simulink model "spwm_single_phase"  (R2020a)
settings: Solver=VariableStepAuto  StartTime=0.0  StopTime=1  RelTol=1e-3
libraries: simulink x16, powerlib_meascontrol x1, powerlib x1
settings Model: Creator=Junaed  LastModifiedBy=Junaed

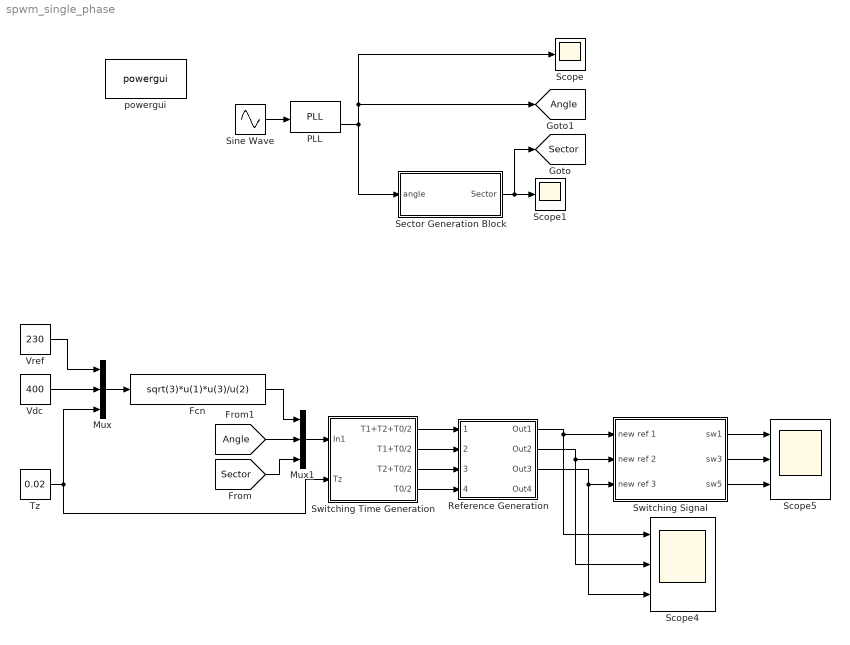
== system spwm_single_phase ==
  Fcn : Fcn  Expr=sqrt(3)*u(1)*u(3)/u(2)
  Mux : Mux  Inputs=3
  Mux1 : Mux  Inputs=3
  PLL : powerlib_meascontrol/PLL/PLL  Fmin=45  Par_Init=[0, 60]  ParK=[180, 3200, 1]  TcD=1e-4  MaxRateChangeFreq=12  FilterCutOffFreq=25  Ts=0  AGC=on
      settings: SourceProductBaseCode=PS
  Reference Generation : Subsystem
  Scope : Scope
  Scope1 : Scope
  Scope4 : Scope  NumInputPorts=3
  Scope5 : Scope  NumInputPorts=3
  Sector Generation Block : Subsystem
  Sine Wave : Sin  Frequency=2*pi*50  SampleTime=0
  "Switching Signal " : Subsystem
  Switching Time Generation : Subsystem
  Tz : Constant  Value=0.02
  Vdc : Constant  Value=400
  Vref : Constant  Value=230
  powergui : powerlib/powergui  Priority=1  SimulationMode=Continuous  SampleTime=50e-6  frequency=60  Iterations=50  frequencyindice=60  Pbase=100e6  ErrMax=1e-4  UnitsV=kV  UnitsW=MW  buscounter=0  FunctionMessages=off  echomessages=off  EnableUseOfTLC=off  CurrentSourceSwitches=off  DisableSnubberDevices=off  DisableRonSwitches=off  DisableVfSwitches=off  DisplayEquations=off  AutomaticDiscreteSolvers=off  SolverType=Tustin/Backward Euler (TBE)  Interpol=off  ExternalGateDelay=off  methode=off  Ts=100  x0status=blocks  SPID=on  SwTol=0  HookPort=off  NonlinearTolerance=1e-4  nMaxIteration=100  ContinueOnMaxIteration=off  RestoreLinks=warning  ResistiveCurrentMeasurement=off  Frange=[0:2:500]  Ylog=off  Xlog=on  ShowGrid=off  save=off  variable=ZData  structure=0  ZoomFFT=off  StartTime=0.0  cycles=1  DisplayStyle=1  fundamental=60  FreqAxis=off  MaxFrequency=1000  frequencyindicesteady=1  RmsSteady=1  display=off
  tag scope: Angle=global, Sector=global
  wires:
  Vref/1 -> Mux/1
  Vdc/1 -> Mux/2
  Tz/1 -> Switching Time Generation/2(Tz), Mux/3
  Mux/1 -> Fcn/1
  Fcn/1 -> Mux1/1
  [Angle] -> Mux1/2
  [Sector] -> Mux1/3
  "Switching Signal "/1(sw1) -> Scope5/1
  "Switching Signal "/2(sw3) -> Scope5/2
  "Switching Signal "/3(sw5) -> Scope5/3
  Mux1/1 -> Switching Time Generation/1(In1)
  Reference Generation/2(Out2) -> "Switching Signal "/2(new ref 2), Scope4/2
  Reference Generation/1(Out1) -> "Switching Signal "/1(new ref 1), Scope4/1
  Switching Time Generation/1(T1+T2+T0/2) -> Reference Generation/1(1)
  Switching Time Generation/2(T1+T0/2) -> Reference Generation/2(2)
  Switching Time Generation/3(T2+T0/2) -> Reference Generation/3(3)
  Switching Time Generation/4(T0/2) -> Reference Generation/4(4)
  PLL/2 -> Sector Generation Block/1(angle), Scope/1, [Angle]
  Sine Wave/1 -> PLL/1
  Sector Generation Block/1(Sector) -> [Sector], Scope1/1
  Reference Generation/3(Out3) -> "Switching Signal "/3(new ref 3), Scope4/3

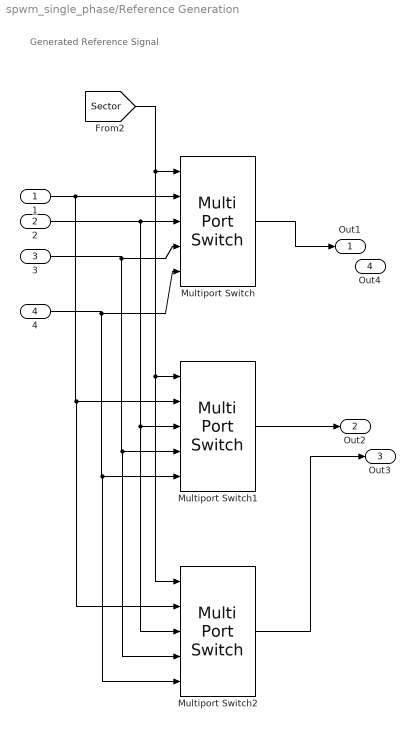
== system spwm_single_phase/Reference Generation ==
  note: Generated Reference Signal
  1 : Inport
  2 : Inport  Port=2
  3 : Inport  Port=3
  4 : Inport  Port=4
  Multiport Switch : MultiPortSwitch  DataPortOrder=Specify indices  Inputs=4  DataPortIndices={[1,6],2,5,[3,4]}
  Multiport Switch1 : MultiPortSwitch  DataPortOrder=Specify indices  Inputs=4  DataPortIndices={[2,3],4,1,[5,6]}
  Multiport Switch2 : MultiPortSwitch  DataPortOrder=Specify indices  Inputs=4  DataPortIndices={[4,5],6,3,[1,2]}
  Out1 : Outport
  Out2 : Outport  Port=2
  Out3 : Outport  Port=3
  Out4 : Outport  Port=4
  wires:
  Multiport Switch2/1 -> Out3/1
  2/1 -> Multiport Switch2/3, Multiport Switch1/3, Multiport Switch/3
  3/1 -> Multiport Switch2/4, Multiport Switch1/4, Multiport Switch/4
  [Sector] -> Multiport Switch2/1, Multiport Switch1/1, Multiport Switch/1
  1/1 -> Multiport Switch2/2, Multiport Switch1/2, Multiport Switch/2
  Multiport Switch/1 -> Out1/1
  Multiport Switch1/1 -> Out2/1
  4/1 -> Multiport Switch2/5, Multiport Switch1/5, Multiport Switch/5

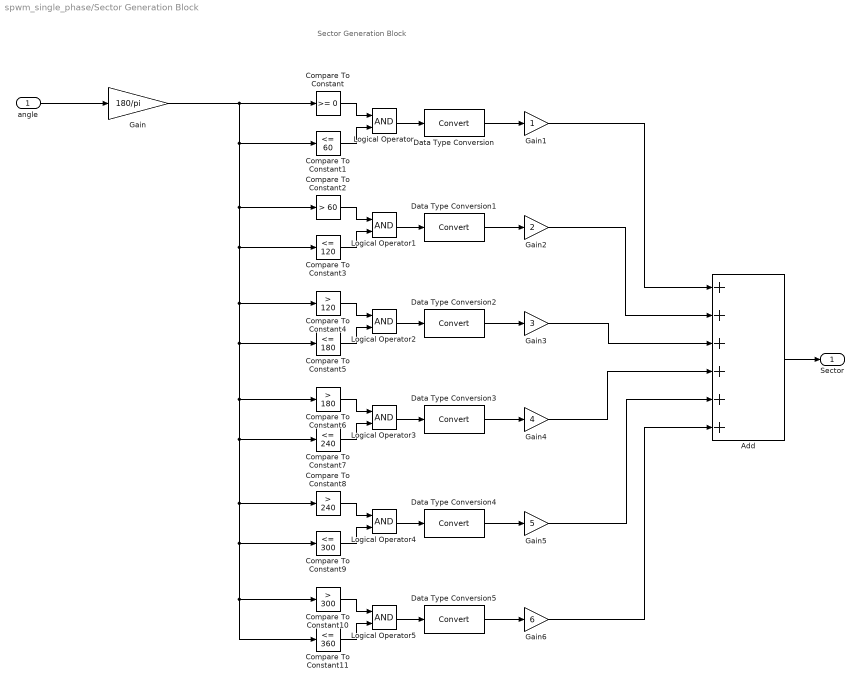
== system spwm_single_phase/Sector Generation Block ==
  note: Sector Generation Block
  angle : Inport
  Add : Sum  Inputs=++++++
  Compare To Constant : simulink/Logic and Bit Operations/Compare To Constant  relop=>=  const=0  OutDataTypeStr=boolean
  Compare To Constant1 : simulink/Logic and Bit Operations/Compare To Constant  relop=<=  const=60  OutDataTypeStr=boolean
  Compare To Constant10 : simulink/Logic and Bit Operations/Compare To Constant  relop=>  const=300  OutDataTypeStr=boolean
  Compare To Constant11 : simulink/Logic and Bit Operations/Compare To Constant  relop=<=  const=360  OutDataTypeStr=boolean
  Compare To Constant2 : simulink/Logic and Bit Operations/Compare To Constant  relop=>  const=60  OutDataTypeStr=boolean
  Compare To Constant3 : simulink/Logic and Bit Operations/Compare To Constant  relop=<=  const=120  OutDataTypeStr=boolean
  Compare To Constant4 : simulink/Logic and Bit Operations/Compare To Constant  relop=>  const=120  OutDataTypeStr=boolean
  Compare To Constant5 : simulink/Logic and Bit Operations/Compare To Constant  relop=<=  const=180  OutDataTypeStr=boolean
  Compare To Constant6 : simulink/Logic and Bit Operations/Compare To Constant  relop=>  const=180  OutDataTypeStr=boolean
  Compare To Constant7 : simulink/Logic and Bit Operations/Compare To Constant  relop=<=  const=240  OutDataTypeStr=boolean
  Compare To Constant8 : simulink/Logic and Bit Operations/Compare To Constant  relop=>  const=240  OutDataTypeStr=boolean
  Compare To Constant9 : simulink/Logic and Bit Operations/Compare To Constant  relop=<=  const=300  OutDataTypeStr=boolean
  Data Type Conversion{,1..5} (6 alike) : DataTypeConversion
  Gain : Gain  Gain=180/pi
  Gain1 : Gain
  Gain2 : Gain  Gain=2
  Gain3 : Gain  Gain=3
  Gain4 : Gain  Gain=4
  Gain5 : Gain  Gain=5
  Gain6 : Gain  Gain=6
  Logical Operator{,1..5} (6 alike) : Logic  AllPortsSameDT=off  OutDataTypeStr=boolean
  Sector : Outport
  wires:
  angle/1 -> Gain/1
  Compare To Constant/1 -> Logical Operator/1
  Compare To Constant1/1 -> Logical Operator/2
  Logical Operator/1 -> Data Type Conversion/1
  Data Type Conversion/1 -> Gain1/1
  Compare To Constant2/1 -> Logical Operator1/1
  Compare To Constant3/1 -> Logical Operator1/2
  Logical Operator1/1 -> Data Type Conversion1/1
  Data Type Conversion1/1 -> Gain2/1
  Compare To Constant4/1 -> Logical Operator2/1
  Compare To Constant5/1 -> Logical Operator2/2
  Logical Operator2/1 -> Data Type Conversion2/1
  Data Type Conversion2/1 -> Gain3/1
  Compare To Constant6/1 -> Logical Operator3/1
  Compare To Constant7/1 -> Logical Operator3/2
  Logical Operator3/1 -> Data Type Conversion3/1
  Data Type Conversion3/1 -> Gain4/1
  Compare To Constant8/1 -> Logical Operator4/1
  Compare To Constant9/1 -> Logical Operator4/2
  Logical Operator4/1 -> Data Type Conversion4/1
  Data Type Conversion4/1 -> Gain5/1
  Compare To Constant10/1 -> Logical Operator5/1
  Compare To Constant11/1 -> Logical Operator5/2
  Logical Operator5/1 -> Data Type Conversion5/1
  Gain/1 -> Compare To Constant2/1, Compare To Constant3/1, Compare To Constant4/1, Compare To Constant5/1, Compare To Constant6/1, Compare To Constant7/1, Compare To Constant8/1, Compare To Constant9/1, Compare To Constant10/1, Compare To Constant11/1, Compare To Constant1/1, Compare To Constant/1
  Data Type Conversion5/1 -> Gain6/1
  Gain1/1 -> Add/1
  Gain2/1 -> Add/2
  Gain3/1 -> Add/3
  Gain4/1 -> Add/4
  Gain5/1 -> Add/5
  Gain6/1 -> Add/6
  Add/1 -> Sector/1

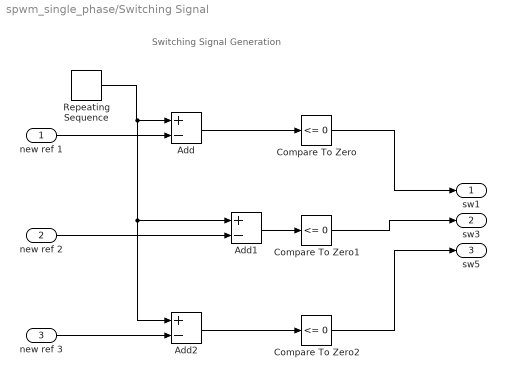
== system spwm_single_phase/Switching Signal  ==
  note: Switching Signal Generation
  new ref 1 : Inport
  new ref 2 : Inport  Port=2
  new ref 3 : Inport  Port=3
  Add : Sum  Inputs=+-
  Add1 : Sum  Inputs=+-
  Add2 : Sum  Inputs=+-
  Compare To Zero : simulink/Logic and Bit Operations/Compare To Zero  relop=<=  OutDataTypeStr=boolean
  Compare To Zero1 : simulink/Logic and Bit Operations/Compare To Zero  relop=<=  OutDataTypeStr=boolean
  Compare To Zero2 : simulink/Logic and Bit Operations/Compare To Zero  relop=<=  OutDataTypeStr=boolean
  Repeating Sequence : simulink/Sources/Repeating Sequence  rep_seq_t=[0 0.001]  rep_seq_y=[0 0.02]
  sw1 : Outport
  sw3 : Outport  Port=2
  sw5 : Outport  Port=3
  wires:
  Repeating Sequence/1 -> Add2/1, Add1/1, Add/1
  new ref 2/1 -> Add1/2
  Add2/1 -> Compare To Zero2/1
  Add1/1 -> Compare To Zero1/1
  new ref 3/1 -> Add2/2
  Add/1 -> Compare To Zero/1
  Compare To Zero1/1 -> sw3/1
  Compare To Zero/1 -> sw1/1
  Compare To Zero2/1 -> sw5/1
  new ref 1/1 -> Add/2

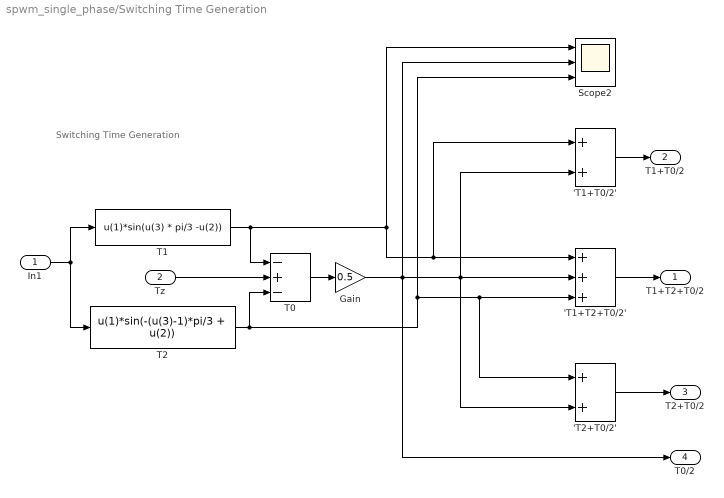
== system spwm_single_phase/Switching Time Generation ==
  note: Switching Time Generation
  In1 : Inport
  Tz : Inport  Port=2
  'T1+T0/2' : Sum
  'T1+T2+T0/2' : Sum  Inputs=+++
  'T2+T0/2' : Sum
  Gain : Gain  Gain=0.5
  Scope2 : Scope  NumInputPorts=3
  T0 : Sum  Inputs=-+-
  T1 : Fcn  Expr=u(1)*sin(u(3) * pi/3 -u(2))
  T2 : Fcn  Expr=u(1)*sin(-(u(3)-1)*pi/3 + u(2))
  T1+T2+T0/2 : Outport
  T1+T0/2 : Outport  Port=2
  T2+T0/2 : Outport  Port=3
  T0/2 : Outport  Port=4
  wires:
  T1/1 -> 'T1+T0/2'/1, 'T1+T2+T0/2'/1, Scope2/1, T0/1
  T2/1 -> 'T2+T0/2'/1, 'T1+T2+T0/2'/3, Scope2/3, T0/3
  In1/1 -> T2/1, T1/1
  'T2+T0/2'/1 -> T2+T0/2/1
  Gain/1 -> T0/2/1, Scope2/2, 'T1+T0/2'/2, 'T2+T0/2'/2, 'T1+T2+T0/2'/2
  'T1+T0/2'/1 -> T1+T0/2/1
  'T1+T2+T0/2'/1 -> T1+T2+T0/2/1
  T0/1 -> Gain/1
  Tz/1 -> T0/2
